simulink model "ds1_inter"  (R2019a)
settings: Solver=ode14x  StartTime=beginTime  StopTime=0.166  FixedStep=1e-4  RelTol=1e-3  EnableMultiTasking=on
model workspace (MAT data in the model file):
  Ankle_L_D = 0.125126243033
  Ankle_L_S = 0.0328154604487
  Ankle_R_D = 0.245807097642
  Ankle_R_S = 0.682954357178
  F_C = 0.06105
  F_H = 0.07
  F_I = 0.00125071180063
  F_L = 0.185
  F_M = 1.13129
  F_W = 0.1
  GRF_HD = 941.037069119
  GRF_HS = 1691.11560066
  GRF_VD = 12300.8672242
  GRF_VS = 71710.3574634
  HAT_I = 3.41998320224
  HAT_L = 0.51264
  HAT_M = 52.89756
  HAT_a = 0.2
  HAT_b = 0.11
  Hip_L_D = 0.0332143791481
  Hip_L_S = 0.0516603438036
  Hip_R_D = 0.145088103411
  Hip_R_S = 0.15911410017
  Knee_L_D = 0.0558982452805
  Knee_L_S = 0.00250387295429
  Knee_R_D = 0.0619293882143
  Knee_R_S = 0.0623339259595
  M : struct (value not decoded)
  Planar_joint_x_p_i = 0
  Planar_joint_x_v_i = 0.571578955042
  Planar_joint_y_p_i = 0
  Planar_joint_y_v_i = 0
  Planar_joint_z_p_i = 0
  Planar_joint_z_w_i = -47.4942945829
  S_I = 0.0556212184297
  S_L = 0.41
  S_M = 3.62793
  S_R1 = 0.035
  S_R2 = 0.0716197243914
  T_I = 0.63371745
  T_L = 0.6
  T_M = 7.802
  T_R1 = 0.0716197243914
  T_R2 = 0.105042262441
  beginTime = 0
  bodymass = 78.02
  lagStanceAnkle = [0 0 0 0 0 0]
  lagStanceKnee = [0 0 0 0 0 0]
  lagSwingAnkle = [0 0 0 0 0 0]
  lagSwingKnee = [0 0 0 0 0 0]
  p_stance_ankle_i = 12.5
  p_stance_hip_i = -24.9413676415
  p_stance_knee_i = -2.50807459996
  p_swing_ankle_i = 4.11757124464
  p_swing_hip_i = 18.3000604838
  p_swing_knee_i = -3.41741510381
  polyfit_stance_ankle = [-863347.977095 222377.922877 -7468.35453889 -9.40558010807 -153.06789694]
  polyfit_stance_hip = [-279786636.688 114363391.625 -15725654.0525 856134.662579 -22930.0516399 481.110496147 63.2694363354]
  polyfit_stance_knee = [-122862314.114 52903969.6705 -7988612.27678 487806.049871 -8969.32141641 330.337585729 -54.0526736443]
  polyfit_swing_ankle = [49510154320.8 -30205907167.6 7312588550.85 -888915044.437 56385922.5861 -1769074.37171 25613.4020917 -113.306543933 -1.03720591697]
  polyfit_swing_hip = [538683495113 -366532634246 101719653645 -14750073882.9 1184454520.37 -50949861.1242 1019832.60417 -6310.84925925 -38.0907282261]
  polyfit_swing_knee = [352478408737 -233011269241 62650744932.5 -8775138187.04 678489689.503 -28060179.8998 545151.783137 -3282.03325692 -26.455631467]
  time = [0 0.00833333333333 0.0166666666667 0.025 0.0333333333333 0.0416666666667 0.05 0.0583333333333 0.0666666666667 0.075 0.0833333333333 0.0916666666667 ... (21 elements, 21x1)]
  w_stance_ankle_i = 4.94863039576
  w_stance_hip_i = 2.61291825988
  w_stance_knee_i = 13.980565237
  w_swing_ankle_i = -56.5478745686
  w_swing_hip_i = 74.5733616561
  w_swing_knee_i = 18.8942606538
symbols that are objects in the model workspace (value not decoded): M
undefined symbols (not defined in the file): X, Y, Z
libraries: nesl_utility x101, sm_lib x68, fl_lib x24, fl_ps_legacy_lib x14, simulink x4
(part 4 of 8)

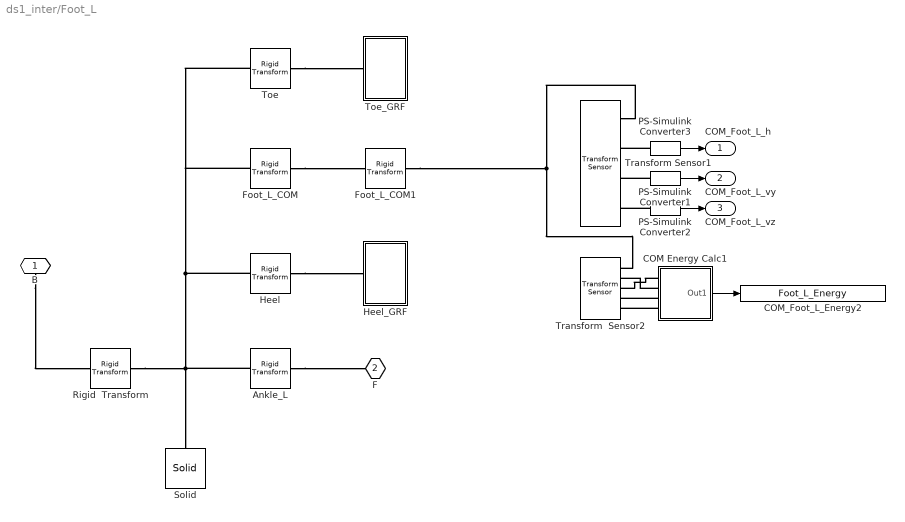
== system ds1_inter/Foot_L ==
  Ankle_L : sm_lib/Frames and Transforms/Rigid Transform  TranslationMethod=StandardAxis  TranslationStandardOffset=F_H  TranslationLengthUnit=m  TranslationStandardAxis=+Y  TranslationCartesianOffset=[0 0 0]  TranslationROffset=0  TranslationROffsetUnits=m  TranslationZOffset=0  TranslationZOffsetUnits=m  TranslationThetaOffset=0  TranslationThetaOffsetUnits=deg  RotationMethod=StandardAxis  RotationAngleUnits=deg  RotationStandardAxis=+Z  RotationAngle=-90  RotationArbitraryAxis=[0 0 1]  FollAlignAxisA=+Z  BaseAlignAxisA=+Z  FollAlignAxisB=+X  BaseAlignAxisB=+Y  RotationSequenceAxes=FollowerAxes  RotationSequence=XYX  RotationSequenceAngles=[0 0 0]  RotationSequenceAnglesUnits=deg  RotationMatrix=[1 0 0; 0 1 0; 0 0 1]
  COM Energy Calc1 : Subsystem
  COM_Foot_L_Energy2 : ToWorkspace  VariableName=Foot_L_Energy  SampleTime=-1
  Foot_L_COM : sm_lib/Frames and Transforms/Rigid Transform  TranslationMethod=StandardAxis  TranslationStandardOffset=(1/3)*F_H  TranslationLengthUnit=m  TranslationStandardAxis=+X  TranslationCartesianOffset=[0 0 0]  TranslationROffset=0  TranslationROffsetUnits=m  TranslationZOffset=0  TranslationZOffsetUnits=m  TranslationThetaOffset=0  TranslationThetaOffsetUnits=deg  RotationMethod=None  RotationAngleUnits=deg  RotationStandardAxis=+X  RotationAngle=0  RotationArbitraryAxis=[0 0 1]  FollAlignAxisA=+X  BaseAlignAxisA=+Z  FollAlignAxisB=+Y  BaseAlignAxisB=+X  RotationSequenceAxes=FollowerAxes  RotationSequence=XYX  RotationSequenceAngles=[0 0 0]  RotationSequenceAnglesUnits=deg  RotationMatrix=[1 0 0; 0 1 0; 0 0 1]
      settings: AttributesFormatString=|
      | {%<RotationStandardAxis>} %<RotationAngle> [%<RotationAngleUnits>]
      | {%<TranslationStandardAxis>} %<TranslationStandardOffset> [%<TranslationLengthUnit>]
  Foot_L_COM1 : sm_lib/Frames and Transforms/Rigid Transform  TranslationMethod=StandardAxis  TranslationStandardOffset=F_H/2  TranslationLengthUnit=m  TranslationStandardAxis=+Y  TranslationCartesianOffset=[0 0 0]  TranslationROffset=0  TranslationROffsetUnits=m  TranslationZOffset=0  TranslationZOffsetUnits=m  TranslationThetaOffset=0  TranslationThetaOffsetUnits=deg  RotationMethod=None  RotationAngleUnits=deg  RotationStandardAxis=+X  RotationAngle=(F_L-F_C)/2  RotationArbitraryAxis=[0 0 1]  FollAlignAxisA=+X  BaseAlignAxisA=+Z  FollAlignAxisB=+Y  BaseAlignAxisB=+X  RotationSequenceAxes=FollowerAxes  RotationSequence=XYX  RotationSequenceAngles=[0 0 0]  RotationSequenceAnglesUnits=deg  RotationMatrix=[1 0 0; 0 1 0; 0 0 1]
      settings: AttributesFormatString=|
      | {%<RotationStandardAxis>} %<RotationAngle> [%<RotationAngleUnits>]
      | {%<TranslationStandardAxis>} %<TranslationStandardOffset> [%<TranslationLengthUnit>]
  Heel : sm_lib/Frames and Transforms/Rigid Transform  TranslationMethod=StandardAxis  TranslationStandardOffset=F_C  TranslationLengthUnit=m  TranslationStandardAxis=-X  TranslationCartesianOffset=[0 0 0]  TranslationROffset=0  TranslationROffsetUnits=m  TranslationZOffset=0  TranslationZOffsetUnits=m  TranslationThetaOffset=0  TranslationThetaOffsetUnits=deg  RotationMethod=AlignedAxes  RotationAngleUnits=deg  RotationStandardAxis=+Z  RotationAngle=0  RotationArbitraryAxis=[0 0 1]  FollAlignAxisA=+X  BaseAlignAxisA=+Z  FollAlignAxisB=+Y  BaseAlignAxisB=+X  RotationSequenceAxes=FollowerAxes  RotationSequence=XYX  RotationSequenceAngles=[0 0 0]  RotationSequenceAnglesUnits=deg  RotationMatrix=[1 0 0; 0 1 0; 0 0 1]
  Heel_GRF : Subsystem
  PS-Simulink Converter1 : nesl_utility/PS-Simulink Converter  PhysicalDomain=network_engine_domain  SubClassName=ps_output  LeftPortType=input  RightPortType=output  PseudoPeriodic=off  Frequencies=[]  Unit=1  AffineConversion=off
  PS-Simulink Converter2 : nesl_utility/PS-Simulink Converter  PhysicalDomain=network_engine_domain  SubClassName=ps_output  LeftPortType=input  RightPortType=output  PseudoPeriodic=off  Frequencies=[]  Unit=1  AffineConversion=off
  PS-Simulink Converter3 : nesl_utility/PS-Simulink Converter  PhysicalDomain=network_engine_domain  SubClassName=ps_output  LeftPortType=input  RightPortType=output  PseudoPeriodic=off  Frequencies=[]  Unit=1  AffineConversion=off
  Rigid  Transform : sm_lib/Frames and Transforms/Rigid Transform  TranslationMethod=None  TranslationStandardOffset=T_R2  TranslationLengthUnit=m  TranslationStandardAxis=+Z  TranslationCartesianOffset=[0 0 0]  TranslationROffset=0  TranslationROffsetUnits=m  TranslationZOffset=0  TranslationZOffsetUnits=m  TranslationThetaOffset=0  TranslationThetaOffsetUnits=deg  RotationMethod=AlignedAxes  RotationAngleUnits=deg  RotationStandardAxis=+Z  RotationAngle=0  RotationArbitraryAxis=[0 0 1]  FollAlignAxisA=+X  BaseAlignAxisA=+Z  FollAlignAxisB=+Z  BaseAlignAxisB=+Y  RotationSequenceAxes=FollowerAxes  RotationSequence=XYX  RotationSequenceAngles=[0 0 0]  RotationSequenceAnglesUnits=deg  RotationMatrix=[1 0 0; 0 1 0; 0 0 1]
  Solid : sm_lib/Body Elements/Solid  InertiaType=Custom  Mass=F_M  MassUnits=kg  CenterOfMass=[(F_L-F_C)/2, F_H/2, 0]  CenterOfMassUnits=m  MomentsOfInertia=[0.001 0.001 F_I]  MomentsOfInertiaUnits=kg*m^2  ProductsOfInertia=[0 0 0]  ProductsOfInertiaUnits=kg*m^2  BasedOnType=Density  Density=0  DensityUnits=kg/(m^3)  DoExposeReferenceFrame=on  SerializedFrames=<Frames/>  GraphicType=FromGeometry  MarkerShape=Sphere  MarkerSize=10  MarkerSizeUnits=m  GraphicVisPropType=SimpleVisualProperties  GraphicDiffuseColor=[0.0 0.4 1.0]  GraphicSpecularColor=[0.5 0.5 0.5 1.0]  GraphicAmbientColor=[0.15 0.15 0.15 1.0]  GraphicEmissiveColor=[0.0 0.0 0.0 1.0]  GraphicShininess=75  GraphicOpacity=1.0  GeometryShape=GeneralExtrusion  RectangleSize=[1 1]  RectangleSizeUnits=m  BrickDimensions=[1 1 1]  BrickDimensionUnits=m  CylinderRadius=1  CylinderRadiusUnits=m  CylinderLength=1  CylinderLengthUnits=m  SphereRadius=1  SphereRadiusUnits=m  EllipsoidRadii=[1 1 1]  EllipsoidRadiiUnits=m  ExtrusionCrossSection=F_cross_section  ExtrusionCrossSectionUnits=m  ExtrusionLength=F_W  ExtrusionLengthUnits=m  PolygonNumSides=3  PolygonOuterRadius=1  PolygonOuterRadiusUnits=m  ExtGeomFileType=STEP  ExtGeomFileUnits=m  RevolutionCrossSection=[1 1; 1 -1; 2 -1; 2 1]  RevolutionCrossSectionUnits=m  RevolutionExtent=Full  RevolutionAngle=180  RevolutionAngleUnits=deg
  Toe : sm_lib/Frames and Transforms/Rigid Transform  TranslationMethod=StandardAxis  TranslationStandardOffset=F_L-F_C  TranslationLengthUnit=m  TranslationStandardAxis=+X  TranslationCartesianOffset=[0 0 0]  TranslationROffset=0  TranslationROffsetUnits=m  TranslationZOffset=0  TranslationZOffsetUnits=m  TranslationThetaOffset=0  TranslationThetaOffsetUnits=deg  RotationMethod=AlignedAxes  RotationAngleUnits=deg  RotationStandardAxis=+Z  RotationAngle=0  RotationArbitraryAxis=[0 0 1]  FollAlignAxisA=+X  BaseAlignAxisA=+Z  FollAlignAxisB=+Y  BaseAlignAxisB=+X  RotationSequenceAxes=FollowerAxes  RotationSequence=XYX  RotationSequenceAngles=[0 0 0]  RotationSequenceAnglesUnits=deg  RotationMatrix=[1 0 0; 0 1 0; 0 0 1]
  Toe_GRF : Subsystem
  Transform Sensor1 : sm_lib/Frames and Transforms/Transform Sensor  MeasurementFrame=World  SenseAngle=off  SenseAxis=off  SenseAngle1=off  SenseAngle2=off  SenseAngle3=off  SenseQ=off  SenseR=off  SenseOmegaX=off  SenseOmegaY=off  SenseOmegaZ=off  SenseOmega1=off  SenseOmega2=off  SenseOmega3=off  SenseQDot=off  SenseRDot=off  SenseAlphaX=off  SenseAlphaY=off  SenseAlphaZ=off  SenseAlpha1=off  SenseAlpha2=off  SenseAlpha3=off  SenseQDDot=off  SenseRDDot=off  SenseX=off  SenseY=off  SenseZ=on  SenseRad=off  SenseAzim=off  SenseDist=off  SenseInc=off  SenseXDot=off  SenseYDot=on  SenseZDot=on  SenseRadDot=off  SenseAzimDot=off  SenseDistDot=off  SenseIncDot=off  SenseXDDot=off  SenseYDDot=off  SenseZDDot=off  SenseRadDDot=off  SenseAzimDDot=off  SenseDistDDot=off  SenseIncDDot=off
  Transform  Sensor2 : sm_lib/Frames and Transforms/Transform Sensor  MeasurementFrame=World  SenseAngle=off  SenseAxis=off  SenseAngle1=off  SenseAngle2=off  SenseAngle3=off  SenseQ=off  SenseR=off  SenseOmegaX=on  SenseOmegaY=off  SenseOmegaZ=off  SenseOmega1=off  SenseOmega2=off  SenseOmega3=off  SenseQDot=off  SenseRDot=off  SenseAlphaX=off  SenseAlphaY=off  SenseAlphaZ=off  SenseAlpha1=off  SenseAlpha2=off  SenseAlpha3=off  SenseQDDot=off  SenseRDDot=off  SenseX=off  SenseY=off  SenseZ=on  SenseRad=off  SenseAzim=off  SenseDist=off  SenseInc=off  SenseXDot=off  SenseYDot=on  SenseZDot=on  SenseRadDot=off  SenseAzimDot=off  SenseDistDot=off  SenseIncDot=off  SenseXDDot=off  SenseYDDot=off  SenseZDDot=off  SenseRadDDot=off  SenseAzimDDot=off  SenseDistDDot=off  SenseIncDDot=off
  B : PMIOPort  Side=Right
  F : PMIOPort  Port=2  Side=Left
  " COM_Foot_L_h" : Outport
  " COM_Foot_L_vy" : Outport  Port=2
  " COM_Foot_L_vz" : Outport  Port=3
  wires:
  COM Energy Calc1/1(Out1) -> COM_Foot_L_Energy2/1
  PS-Simulink Converter1/1 -> " COM_Foot_L_vy"/1
  PS-Simulink Converter3/1 -> " COM_Foot_L_h"/1
  PS-Simulink Converter2/1 -> " COM_Foot_L_vz"/1
  connections:
  B/RConn1 -- Rigid  Transform/RConn1
  Rigid  Transform/LConn1 -- Ankle_L/LConn1 -- Foot_L_COM/LConn1 -- Toe/LConn1 -- Heel/LConn1 -- Solid/RConn1
  Ankle_L/RConn1 -- F/RConn1
  Toe/RConn1 -- Toe_GRF/LConn1
  Heel/RConn1 -- Heel_GRF/LConn1
  Transform Sensor1/RConn1 -- Transform  Sensor2/RConn1 -- Foot_L_COM1/RConn1
  COM Energy Calc1/LConn2 -- Transform  Sensor2/RConn2
  COM Energy Calc1/LConn4 -- Transform  Sensor2/RConn5
  PS-Simulink Converter1/LConn1 -- Transform Sensor1/RConn3
  COM Energy Calc1/LConn1 -- Transform  Sensor2/RConn3
  PS-Simulink Converter2/LConn1 -- Transform Sensor1/RConn4
  COM Energy Calc1/LConn3 -- Transform  Sensor2/RConn4
  PS-Simulink Converter3/LConn1 -- Transform Sensor1/RConn2
  Foot_L_COM/RConn1 -- Foot_L_COM1/LConn1

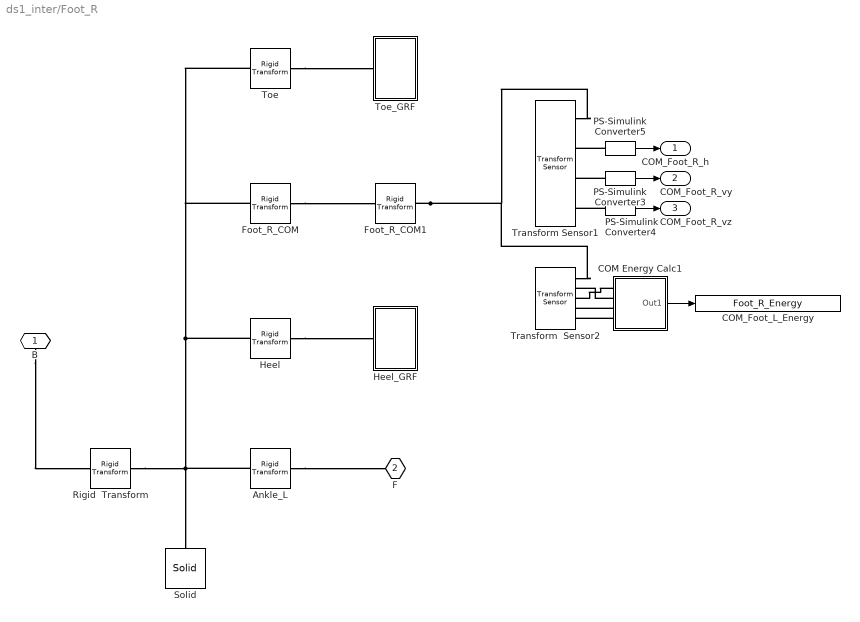
== system ds1_inter/Foot_R ==
  Ankle_L : sm_lib/Frames and Transforms/Rigid Transform  TranslationMethod=StandardAxis  TranslationStandardOffset=F_H  TranslationLengthUnit=m  TranslationStandardAxis=+Y  TranslationCartesianOffset=[0 0 0]  TranslationROffset=0  TranslationROffsetUnits=m  TranslationZOffset=0  TranslationZOffsetUnits=m  TranslationThetaOffset=0  TranslationThetaOffsetUnits=deg  RotationMethod=StandardAxis  RotationAngleUnits=deg  RotationStandardAxis=+Z  RotationAngle=-90  RotationArbitraryAxis=[0 0 1]  FollAlignAxisA=+Z  BaseAlignAxisA=+Z  FollAlignAxisB=+X  BaseAlignAxisB=+Y  RotationSequenceAxes=FollowerAxes  RotationSequence=XYX  RotationSequenceAngles=[0 0 0]  RotationSequenceAnglesUnits=deg  RotationMatrix=[1 0 0; 0 1 0; 0 0 1]
      settings: AttributesFormatString=|
      | {%<RotationStandardAxis>} %<RotationAngle> [%<RotationAngleUnits>]
      | {%<TranslationStandardAxis>} %<TranslationStandardOffset> [%<TranslationLengthUnit>]
  COM Energy Calc1 : Subsystem
  COM_Foot_L_Energy : ToWorkspace  VariableName=Foot_R_Energy  SampleTime=-1
  Foot_R_COM : sm_lib/Frames and Transforms/Rigid Transform  TranslationMethod=StandardAxis  TranslationStandardOffset=(1/3)*F_H  TranslationLengthUnit=m  TranslationStandardAxis=+X  TranslationCartesianOffset=[0 0 0]  TranslationROffset=0  TranslationROffsetUnits=m  TranslationZOffset=0  TranslationZOffsetUnits=m  TranslationThetaOffset=0  TranslationThetaOffsetUnits=deg  RotationMethod=None  RotationAngleUnits=deg  RotationStandardAxis=+X  RotationAngle=0  RotationArbitraryAxis=[0 0 1]  FollAlignAxisA=+X  BaseAlignAxisA=+Z  FollAlignAxisB=+Y  BaseAlignAxisB=+X  RotationSequenceAxes=FollowerAxes  RotationSequence=XYX  RotationSequenceAngles=[0 0 0]  RotationSequenceAnglesUnits=deg  RotationMatrix=[1 0 0; 0 1 0; 0 0 1]
      settings: AttributesFormatString=|
      | {%<RotationStandardAxis>} %<RotationAngle> [%<RotationAngleUnits>]
      | {%<TranslationStandardAxis>} %<TranslationStandardOffset> [%<TranslationLengthUnit>]
  Foot_R_COM1 : sm_lib/Frames and Transforms/Rigid Transform  TranslationMethod=StandardAxis  TranslationStandardOffset=F_H/2  TranslationLengthUnit=m  TranslationStandardAxis=+Y  TranslationCartesianOffset=[0 0 0]  TranslationROffset=0  TranslationROffsetUnits=m  TranslationZOffset=0  TranslationZOffsetUnits=m  TranslationThetaOffset=0  TranslationThetaOffsetUnits=deg  RotationMethod=None  RotationAngleUnits=deg  RotationStandardAxis=+X  RotationAngle=(F_L-F_C)/2  RotationArbitraryAxis=[0 0 1]  FollAlignAxisA=+X  BaseAlignAxisA=+Z  FollAlignAxisB=+Y  BaseAlignAxisB=+X  RotationSequenceAxes=FollowerAxes  RotationSequence=XYX  RotationSequenceAngles=[0 0 0]  RotationSequenceAnglesUnits=deg  RotationMatrix=[1 0 0; 0 1 0; 0 0 1]
      settings: AttributesFormatString=|
      | {%<RotationStandardAxis>} %<RotationAngle> [%<RotationAngleUnits>]
      | {%<TranslationStandardAxis>} %<TranslationStandardOffset> [%<TranslationLengthUnit>]
  Heel : sm_lib/Frames and Transforms/Rigid Transform  TranslationMethod=StandardAxis  TranslationStandardOffset=F_C  TranslationLengthUnit=m  TranslationStandardAxis=-X  TranslationCartesianOffset=[0 0 0]  TranslationROffset=0  TranslationROffsetUnits=m  TranslationZOffset=0  TranslationZOffsetUnits=m  TranslationThetaOffset=0  TranslationThetaOffsetUnits=deg  RotationMethod=AlignedAxes  RotationAngleUnits=deg  RotationStandardAxis=+Z  RotationAngle=0  RotationArbitraryAxis=[0 0 1]  FollAlignAxisA=+X  BaseAlignAxisA=+Z  FollAlignAxisB=+Y  BaseAlignAxisB=+X  RotationSequenceAxes=FollowerAxes  RotationSequence=XYX  RotationSequenceAngles=[0 0 0]  RotationSequenceAnglesUnits=deg  RotationMatrix=[1 0 0; 0 1 0; 0 0 1]
      settings: AttributesFormatString=|
      | {%<RotationStandardAxis>} %<RotationAngle> [%<RotationAngleUnits>]
      | {%<TranslationStandardAxis>} %<TranslationStandardOffset> [%<TranslationLengthUnit>]
  Heel_GRF : Subsystem
  PS-Simulink Converter3 : nesl_utility/PS-Simulink Converter  PhysicalDomain=network_engine_domain  SubClassName=ps_output  LeftPortType=input  RightPortType=output  PseudoPeriodic=off  Frequencies=[]  Unit=1  AffineConversion=off
  PS-Simulink Converter4 : nesl_utility/PS-Simulink Converter  PhysicalDomain=network_engine_domain  SubClassName=ps_output  LeftPortType=input  RightPortType=output  PseudoPeriodic=off  Frequencies=[]  Unit=1  AffineConversion=off
  PS-Simulink Converter5 : nesl_utility/PS-Simulink Converter  PhysicalDomain=network_engine_domain  SubClassName=ps_output  LeftPortType=input  RightPortType=output  PseudoPeriodic=off  Frequencies=[]  Unit=1  AffineConversion=off
  Rigid  Transform : sm_lib/Frames and Transforms/Rigid Transform  TranslationMethod=StandardAxis  TranslationStandardOffset=T_R2  TranslationLengthUnit=m  TranslationStandardAxis=+Z  TranslationCartesianOffset=[0 0 0]  TranslationROffset=0  TranslationROffsetUnits=m  TranslationZOffset=0  TranslationZOffsetUnits=m  TranslationThetaOffset=0  TranslationThetaOffsetUnits=deg  RotationMethod=AlignedAxes  RotationAngleUnits=deg  RotationStandardAxis=+Z  RotationAngle=0  RotationArbitraryAxis=[0 0 1]  FollAlignAxisA=+X  BaseAlignAxisA=+Z  FollAlignAxisB=+Z  BaseAlignAxisB=+Y  RotationSequenceAxes=FollowerAxes  RotationSequence=XYX  RotationSequenceAngles=[0 0 0]  RotationSequenceAnglesUnits=deg  RotationMatrix=[1 0 0; 0 1 0; 0 0 1]
      settings: AttributesFormatString=|
      | {%<RotationStandardAxis>} %<RotationAngle> [%<RotationAngleUnits>]
      | {%<TranslationStandardAxis>} %<TranslationStandardOffset> [%<TranslationLengthUnit>]
  Solid : sm_lib/Body Elements/Solid  InertiaType=Custom  Mass=F_M  MassUnits=kg  CenterOfMass=[(F_L-F_C)/2, F_H/2, 0]  CenterOfMassUnits=m  MomentsOfInertia=[0.001 0.001 F_I]  MomentsOfInertiaUnits=kg*m^2  ProductsOfInertia=[0 0 0]  ProductsOfInertiaUnits=kg*m^2  BasedOnType=Density  Density=0  DensityUnits=kg/(m^3)  DoExposeReferenceFrame=on  SerializedFrames=<Frames/>  GraphicType=FromGeometry  MarkerShape=Sphere  MarkerSize=10  MarkerSizeUnits=m  GraphicVisPropType=SimpleVisualProperties  GraphicDiffuseColor=[0.0 0.4 1.0]  GraphicSpecularColor=[0.5 0.5 0.5 1.0]  GraphicAmbientColor=[0.15 0.15 0.15 1.0]  GraphicEmissiveColor=[0.0 0.0 0.0 1.0]  GraphicShininess=75  GraphicOpacity=1.0  GeometryShape=GeneralExtrusion  RectangleSize=[1 1]  RectangleSizeUnits=m  BrickDimensions=[1 1 1]  BrickDimensionUnits=m  CylinderRadius=1  CylinderRadiusUnits=m  CylinderLength=1  CylinderLengthUnits=m  SphereRadius=1  SphereRadiusUnits=m  EllipsoidRadii=[1 1 1]  EllipsoidRadiiUnits=m  ExtrusionCrossSection=F_cross_section  ExtrusionCrossSectionUnits=m  ExtrusionLength=F_W  ExtrusionLengthUnits=m  PolygonNumSides=3  PolygonOuterRadius=1  PolygonOuterRadiusUnits=m  ExtGeomFileType=STEP  ExtGeomFileUnits=m  RevolutionCrossSection=[1 1; 1 -1; 2 -1; 2 1]  RevolutionCrossSectionUnits=m  RevolutionExtent=Full  RevolutionAngle=180  RevolutionAngleUnits=deg
  Toe : sm_lib/Frames and Transforms/Rigid Transform  TranslationMethod=StandardAxis  TranslationStandardOffset=F_L-F_C  TranslationLengthUnit=m  TranslationStandardAxis=+X  TranslationCartesianOffset=[0 0 0]  TranslationROffset=0  TranslationROffsetUnits=m  TranslationZOffset=0  TranslationZOffsetUnits=m  TranslationThetaOffset=0  TranslationThetaOffsetUnits=deg  RotationMethod=AlignedAxes  RotationAngleUnits=deg  RotationStandardAxis=+Z  RotationAngle=0  RotationArbitraryAxis=[0 0 1]  FollAlignAxisA=+X  BaseAlignAxisA=+Z  FollAlignAxisB=+Y  BaseAlignAxisB=+X  RotationSequenceAxes=FollowerAxes  RotationSequence=XYX  RotationSequenceAngles=[0 0 0]  RotationSequenceAnglesUnits=deg  RotationMatrix=[1 0 0; 0 1 0; 0 0 1]
      settings: AttributesFormatString=|
      | {%<RotationStandardAxis>} %<RotationAngle> [%<RotationAngleUnits>]
      | {%<TranslationStandardAxis>} %<TranslationStandardOffset> [%<TranslationLengthUnit>]
  "Toe_GRF " : Subsystem
  Transform Sensor1 : sm_lib/Frames and Transforms/Transform Sensor  MeasurementFrame=World  SenseAngle=off  SenseAxis=off  SenseAngle1=off  SenseAngle2=off  SenseAngle3=off  SenseQ=off  SenseR=off  SenseOmegaX=off  SenseOmegaY=off  SenseOmegaZ=off  SenseOmega1=off  SenseOmega2=off  SenseOmega3=off  SenseQDot=off  SenseRDot=off  SenseAlphaX=off  SenseAlphaY=off  SenseAlphaZ=off  SenseAlpha1=off  SenseAlpha2=off  SenseAlpha3=off  SenseQDDot=off  SenseRDDot=off  SenseX=off  SenseY=off  SenseZ=on  SenseRad=off  SenseAzim=off  SenseDist=off  SenseInc=off  SenseXDot=off  SenseYDot=on  SenseZDot=on  SenseRadDot=off  SenseAzimDot=off  SenseDistDot=off  SenseIncDot=off  SenseXDDot=off  SenseYDDot=off  SenseZDDot=off  SenseRadDDot=off  SenseAzimDDot=off  SenseDistDDot=off  SenseIncDDot=off
  Transform  Sensor2 : sm_lib/Frames and Transforms/Transform Sensor  MeasurementFrame=World  SenseAngle=off  SenseAxis=off  SenseAngle1=off  SenseAngle2=off  SenseAngle3=off  SenseQ=off  SenseR=off  SenseOmegaX=on  SenseOmegaY=off  SenseOmegaZ=off  SenseOmega1=off  SenseOmega2=off  SenseOmega3=off  SenseQDot=off  SenseRDot=off  SenseAlphaX=off  SenseAlphaY=off  SenseAlphaZ=off  SenseAlpha1=off  SenseAlpha2=off  SenseAlpha3=off  SenseQDDot=off  SenseRDDot=off  SenseX=off  SenseY=off  SenseZ=on  SenseRad=off  SenseAzim=off  SenseDist=off  SenseInc=off  SenseXDot=off  SenseYDot=on  SenseZDot=on  SenseRadDot=off  SenseAzimDot=off  SenseDistDot=off  SenseIncDot=off  SenseXDDot=off  SenseYDDot=off  SenseZDDot=off  SenseRadDDot=off  SenseAzimDDot=off  SenseDistDDot=off  SenseIncDDot=off
  B : PMIOPort  Side=Right
  F : PMIOPort  Port=2  Side=Left
  COM_Foot_R_h : Outport
  COM_Foot_R_vy : Outport  Port=2
  COM_Foot_R_vz : Outport  Port=3
  wires:
  PS-Simulink Converter5/1 -> COM_Foot_R_h/1
  PS-Simulink Converter4/1 -> COM_Foot_R_vz/1
  COM Energy Calc1/1(Out1) -> COM_Foot_L_Energy/1
  PS-Simulink Converter3/1 -> COM_Foot_R_vy/1
  connections:
  B/RConn1 -- Rigid  Transform/RConn1
  Rigid  Transform/LConn1 -- Ankle_L/LConn1 -- Foot_R_COM/LConn1 -- Toe/LConn1 -- Heel/LConn1 -- Solid/RConn1
  Ankle_L/RConn1 -- F/RConn1
  Heel/RConn1 -- Heel_GRF/LConn1
  Toe/RConn1 -- "Toe_GRF "/LConn1
  Foot_R_COM1/RConn1 -- Transform  Sensor2/RConn1 -- Transform Sensor1/RConn1
  PS-Simulink Converter5/LConn1 -- Transform Sensor1/RConn2
  COM Energy Calc1/LConn1 -- Transform  Sensor2/RConn3
  COM Energy Calc1/LConn2 -- Transform  Sensor2/RConn2
  COM Energy Calc1/LConn4 -- Transform  Sensor2/RConn5
  COM Energy Calc1/LConn3 -- Transform  Sensor2/RConn4
  PS-Simulink Converter4/LConn1 -- Transform Sensor1/RConn4
  PS-Simulink Converter3/LConn1 -- Transform Sensor1/RConn3
  Foot_R_COM/RConn1 -- Foot_R_COM1/LConn1

== system ds1_inter/HAT ==
  note: %vCOMCal  uses transform sensor to read velocity of COM in y(forward)
      | and z(up) wrt world frame
  Gain : Gain  Gain=180/pi
  PS-Simulink Converter{,1..3} (4 alike) : nesl_utility/PS-Simulink Converter  PhysicalDomain=network_engine_domain  SubClassName=ps_output  LeftPortType=input  RightPortType=output  PseudoPeriodic=off  Frequencies=[]  Unit=1  AffineConversion=off
  PredictedCOMVelocity_y : ToWorkspace  VariableName=PredictedCOMVelocity_y  SampleTime=-1
      settings: MaxDataPoints=1  Decimation=3
  PredictedCOMVelocity_y1 : ToWorkspace  VariableName=PredictedCOMVelocity_z  SampleTime=-1
      settings: MaxDataPoints=1  Decimation=3
  Rigid  Transform : sm_lib/Frames and Transforms/Rigid Transform  TranslationMethod=Cartesian  TranslationStandardOffset=0  TranslationLengthUnit=m  TranslationStandardAxis=+Z  TranslationCartesianOffset=[-T_R2, 0, -HAT_L/2]  TranslationROffset=0  TranslationROffsetUnits=m  TranslationZOffset=0  TranslationZOffsetUnits=m  TranslationThetaOffset=0  TranslationThetaOffsetUnits=deg  RotationMethod=StandardAxis  RotationAngleUnits=deg  RotationStandardAxis=+Y  RotationAngle=90  RotationArbitraryAxis=[0 0 1]  FollAlignAxisA=+X  BaseAlignAxisA=+Y  FollAlignAxisB=+Y  BaseAlignAxisB=+Z  RotationSequenceAxes=FollowerAxes  RotationSequence=XYX  RotationSequenceAngles=[0 0 0]  RotationSequenceAnglesUnits=deg  RotationMatrix=[1 0 0; 0 1 0; 0 0 1]
  Rigid  Transform1 : sm_lib/Frames and Transforms/Rigid Transform  TranslationMethod=Cartesian  TranslationStandardOffset=0  TranslationLengthUnit=m  TranslationStandardAxis=+Z  TranslationCartesianOffset=[T_R2, 0, -HAT_L/2]  TranslationROffset=0  TranslationROffsetUnits=m  TranslationZOffset=0  TranslationZOffsetUnits=m  TranslationThetaOffset=0  TranslationThetaOffsetUnits=deg  RotationMethod=StandardAxis  RotationAngleUnits=deg  RotationStandardAxis=+Y  RotationAngle=90  RotationArbitraryAxis=[0 0 1]  FollAlignAxisA=+X  BaseAlignAxisA=+Y  FollAlignAxisB=+Y  BaseAlignAxisB=+Z  RotationSequenceAxes=FollowerAxes  RotationSequence=XYX  RotationSequenceAngles=[0 0 0]  RotationSequenceAnglesUnits=deg  RotationMatrix=[1 0 0; 0 1 0; 0 0 1]
  Scope : Scope
  Scope1 : Scope
  Scope2 : Scope
  Solid : sm_lib/Body Elements/Solid  InertiaType=Custom  Mass=HAT_M  MassUnits=kg  CenterOfMass=[0 0 .126*HAT_L]  CenterOfMassUnits=m  MomentsOfInertia=[HAT_I .001 .001]  MomentsOfInertiaUnits=kg*m^2  ProductsOfInertia=[0 0 0]  ProductsOfInertiaUnits=kg*m^2  BasedOnType=Density  Density=1000  DensityUnits=kg/(m^3)  DoExposeReferenceFrame=on  SerializedFrames=<Frames/>  GraphicType=FromGeometry  MarkerShape=Sphere  MarkerSize=10  MarkerSizeUnits=m  GraphicVisPropType=SimpleVisualProperties  GraphicDiffuseColor=[0.0 0.4 1.0]  GraphicSpecularColor=[0.5 0.5 0.5 1.0]  GraphicAmbientColor=[0.15 0.15 0.15 1.0]  GraphicEmissiveColor=[0.0 0.0 0.0 1.0]  GraphicShininess=75  GraphicOpacity=1.0  GeometryShape=GeneralExtrusion  RectangleSize=[1 1]  RectangleSizeUnits=m  BrickDimensions=[1 1 1]  BrickDimensionUnits=m  CylinderRadius=1  CylinderRadiusUnits=m  CylinderLength=1  CylinderLengthUnits=m  SphereRadius=1  SphereRadiusUnits=m  EllipsoidRadii=[1 1 1]  EllipsoidRadiiUnits=m  ExtrusionCrossSection=HAT_cross_section  ExtrusionCrossSectionUnits=m  ExtrusionLength=HAT_L  ExtrusionLengthUnits=m  PolygonNumSides=3  PolygonOuterRadius=1  PolygonOuterRadiusUnits=m  ExtGeomFileType=STEP  ExtGeomFileUnits=m  RevolutionCrossSection=[1 1; 1 -1; 2 -1; 2 1]  RevolutionCrossSectionUnits=m  RevolutionExtent=Full  RevolutionAngle=180  RevolutionAngleUnits=deg
  Transform  Sensor : sm_lib/Frames and Transforms/Transform Sensor  MeasurementFrame=World  SenseAngle=on  SenseAxis=off  SenseAngle1=off  SenseAngle2=off  SenseAngle3=off  SenseQ=off  SenseR=off  SenseOmegaX=off  SenseOmegaY=off  SenseOmegaZ=off  SenseOmega1=off  SenseOmega2=off  SenseOmega3=off  SenseQDot=off  SenseRDot=off  SenseAlphaX=off  SenseAlphaY=off  SenseAlphaZ=off  SenseAlpha1=off  SenseAlpha2=off  SenseAlpha3=off  SenseQDDot=off  SenseRDDot=off  SenseX=off  SenseY=off  SenseZ=off  SenseRad=off  SenseAzim=off  SenseDist=off  SenseInc=off  SenseXDot=on  SenseYDot=on  SenseZDot=on  SenseRadDot=off  SenseAzimDot=off  SenseDistDot=off  SenseIncDot=off  SenseXDDot=off  SenseYDDot=off  SenseZDDot=off  SenseRadDDot=off  SenseAzimDDot=off  SenseDistDDot=off  SenseIncDDot=off
  vCOMCal : Subsystem
  B : PMIOPort  Side=Right
  F1 : PMIOPort  Port=2  Side=Left
  F2 : PMIOPort  Port=3  Side=Left
  HAT_position : Outport
  wires:
  PS-Simulink Converter/1 -> Gain/1
  Gain/1 -> HAT_position/1
  PS-Simulink Converter1/1 -> Scope/1
  PS-Simulink Converter2/1 -> Scope1/1
  PS-Simulink Converter3/1 -> Scope2/1
  vCOMCal/2(vCOM_z) -> PredictedCOMVelocity_y1/1
  vCOMCal/1(vCOM_y) -> PredictedCOMVelocity_y/1
  connections:
  B/RConn1 -- Transform  Sensor/RConn1 -- Rigid  Transform1/LConn1 -- Solid/RConn1 -- Rigid  Transform/LConn1
  Rigid  Transform1/RConn1 -- F2/RConn1
  Rigid  Transform/RConn1 -- vCOMCal/LConn1 -- F1/RConn1
  Transform  Sensor/RConn2 -- PS-Simulink Converter/LConn1
  Transform  Sensor/RConn3 -- PS-Simulink Converter1/LConn1
  Transform  Sensor/RConn4 -- PS-Simulink Converter2/LConn1
  Transform  Sensor/RConn5 -- PS-Simulink Converter3/LConn1

== system ds1_inter/Hip_L_Actuation ==
  Clock : Clock
  Gain : Gain  Gain=-1
  Hard_Stop_Hip_L : Subsystem  mask{upper_bound=((125-p_stance_hip_i)*pi)/180, lower_bound=((-30-p_stance_hip_i)*pi)/180, contact_stiffness=1e8, contact_damping=5000, initial_angular_position=0}
      mask prompts: upper_bound "Upper Bound"; lower_bound "Lower Bound"; contact_stiffness "Contact Stiffness"; contact_damping "Contact Damping"; initial_angular_position "Initial Angular Position"
  Hip_D_lookup : Lookup_n-D  NumberOfTableDimensions=1  BreakpointsForDimension1=[-30:.01:125]  Table=[exp(linspace(log(1000),log(.01),1000)), zeros(1,13500),exp(linspace(log(.01),log(1000),1001))]  RndMeth=Simplest  InputSameDT=on
  Hip_S_lookup : Lookup_n-D  NumberOfTableDimensions=1  BreakpointsForDimension1=[-30:.01:125]  Table=[exp(linspace(log(10000),log(.01),1000)), zeros(1,13500),exp(linspace(log(.01),log(10000),1001))]  RndMeth=Simplest  InputSameDT=on
  PS Add : fl_ps_legacy_lib/Legacy Physical Signals/Functions/PS Add
      settings: SourceProductName=Simscape  SourceProductBaseCode=SS
  PS Add1 : fl_ps_legacy_lib/Legacy Physical Signals/Functions/PS Add
      settings: SourceProductName=Simscape  SourceProductBaseCode=SS
  PS Lookup Table (1D) : fl_ps_legacy_lib/Legacy Physical Signals/Lookup Tables/PS Lookup Table (1D)  x=linspace(0,.1667,21)'  f=(-M.stance_hip/1000)*bodymass  interp_method=2  extrap_method=1
      settings: SourceProductName=Simscape  SourceProductBaseCode=SS
  PS-Simulink Converter1 : nesl_utility/PS-Simulink Converter  PhysicalDomain=network_engine_domain  SubClassName=ps_output  LeftPortType=input  RightPortType=output  PseudoPeriodic=off  Frequencies=[]  Unit=1  AffineConversion=off
  PS-Simulink Converter2 : nesl_utility/PS-Simulink Converter  PhysicalDomain=network_engine_domain  SubClassName=ps_output  LeftPortType=input  RightPortType=output  PseudoPeriodic=off  Frequencies=[]  Unit=1  AffineConversion=off
  Product : Product  RndMeth=Zero
  Product1 : Product  RndMeth=Zero
  Simulink-PS Converter : nesl_utility/Simulink-PS Converter  PhysicalDomain=network_engine_domain  SubClassName=ps_input  LeftPortType=input  RightPortType=output  PseudoPeriodic=off  Frequencies=[]  NoiseDistribution=none  NoiseParameters=[]  Unit=1  AffineConversion=off  FilteringAndDerivatives=zero  SimscapeFilterOrder=1  InputFilterTimeConstant=.001  UdotUserProvided=[]
  Simulink-PS Converter1 : nesl_utility/Simulink-PS Converter  PhysicalDomain=network_engine_domain  SubClassName=ps_input  LeftPortType=input  RightPortType=output  PseudoPeriodic=off  Frequencies=[]  NoiseDistribution=none  NoiseParameters=[]  Unit=1  AffineConversion=off  FilteringAndDerivatives=zero  SimscapeFilterOrder=1  InputFilterTimeConstant=.001  UdotUserProvided=[]
  Sum : Sum  Inputs=|++
  rad2deg : Gain  Gain=180/pi
  "rad2deg1 " : Gain  Gain=180/pi
  w : PMIOPort  Side=Right
  t : PMIOPort  Port=2  Side=Left
  q : PMIOPort  Port=3  Side=Right
  wires:
  PS-Simulink Converter1/1 -> "rad2deg1 "/1
  PS-Simulink Converter2/1 -> rad2deg/1
  rad2deg/1 -> Hip_S_lookup/1, Hip_D_lookup/1, Product/2
  Hip_S_lookup/1 -> Product/1
  "rad2deg1 "/1 -> Product1/1
  Product1/1 -> Sum/1
  Product/1 -> Sum/2
  Sum/1 -> Gain/1
  Gain/1 -> Simulink-PS Converter1/1
  Hip_D_lookup/1 -> Product1/2
  Clock/1 -> Simulink-PS Converter/1
  connections:
  w/RConn1 -- PS-Simulink Converter1/LConn1 -- Hard_Stop_Hip_L/LConn1
  Hard_Stop_Hip_L/RConn1 -- PS Add/LConn2
  q/RConn1 -- PS-Simulink Converter2/LConn1
  PS Add1/RConn1 -- t/RConn1
  PS Add/RConn1 -- PS Add1/LConn1
  Simulink-PS Converter1/RConn1 -- PS Add1/LConn2
  PS Lookup Table (1D)/RConn1 -- PS Add/LConn1
  Simulink-PS Converter/RConn1 -- PS Lookup Table (1D)/LConn1

== system ds1_inter/Hip_R_Actuation ==
  Clock : Clock
  Gain : Gain  Gain=-1
  Hard_Stop_Hip_R : Subsystem  mask{upper_bound=((125-p_swing_hip_i)*pi)/180, lower_bound=((-30-p_swing_hip_i)*pi)/180, contact_stiffness=1e8, contact_damping=5000, initial_angular_position=0}
      mask prompts: upper_bound "Upper Bound"; lower_bound "Lower Bound"; contact_stiffness "Contact Stiffness"; contact_damping "Contact Damping"; initial_angular_position "Initial Angular Position"
  Hip_D_lookup : Lookup_n-D  NumberOfTableDimensions=1  BreakpointsForDimension1=[-30:.01:125]  Table=[exp(linspace(log(1000),log(.01),1000)), zeros(1,13500),exp(linspace(log(.01),log(1000),1001))]  RndMeth=Simplest  InputSameDT=on
  Hip_S_lookup : Lookup_n-D  NumberOfTableDimensions=1  BreakpointsForDimension1=[-30:.01:125]  Table=[exp(linspace(log(10000),log(.01),1000)), zeros(1,13500),exp(linspace(log(.01),log(10000),1001))]  RndMeth=Simplest  InputSameDT=on
  PS Add : fl_ps_legacy_lib/Legacy Physical Signals/Functions/PS Add
      settings: SourceProductName=Simscape  SourceProductBaseCode=SS
  PS Add1 : fl_ps_legacy_lib/Legacy Physical Signals/Functions/PS Add
      settings: SourceProductName=Simscape  SourceProductBaseCode=SS
  PS Lookup Table (1D) : fl_ps_legacy_lib/Legacy Physical Signals/Lookup Tables/PS Lookup Table (1D)  x=linspace(0,.1667,21)'  f=(-M.strike_hip/1000)*bodymass  interp_method=2  extrap_method=1
      settings: SourceProductName=Simscape  SourceProductBaseCode=SS
  PS-Simulink Converter1 : nesl_utility/PS-Simulink Converter  PhysicalDomain=network_engine_domain  SubClassName=ps_output  LeftPortType=input  RightPortType=output  PseudoPeriodic=off  Frequencies=[]  Unit=1  AffineConversion=off
  PS-Simulink Converter2 : nesl_utility/PS-Simulink Converter  PhysicalDomain=network_engine_domain  SubClassName=ps_output  LeftPortType=input  RightPortType=output  PseudoPeriodic=off  Frequencies=[]  Unit=1  AffineConversion=off
  Product : Product  RndMeth=Zero
  Product1 : Product  RndMeth=Zero
  Simulink-PS Converter : nesl_utility/Simulink-PS Converter  PhysicalDomain=network_engine_domain  SubClassName=ps_input  LeftPortType=input  RightPortType=output  PseudoPeriodic=off  Frequencies=[]  NoiseDistribution=none  NoiseParameters=[]  Unit=1  AffineConversion=off  FilteringAndDerivatives=zero  SimscapeFilterOrder=1  InputFilterTimeConstant=.001  UdotUserProvided=[]
  Simulink-PS Converter1 : nesl_utility/Simulink-PS Converter  PhysicalDomain=network_engine_domain  SubClassName=ps_input  LeftPortType=input  RightPortType=output  PseudoPeriodic=off  Frequencies=[]  NoiseDistribution=none  NoiseParameters=[]  Unit=1  AffineConversion=off  FilteringAndDerivatives=zero  SimscapeFilterOrder=1  InputFilterTimeConstant=.001  UdotUserProvided=[]
  Sum : Sum  Inputs=|++
  rad2deg : Gain  Gain=180/pi
  "rad2deg1 " : Gain  Gain=180/pi
  w : PMIOPort  Side=Right
  t : PMIOPort  Port=2  Side=Left
  q : PMIOPort  Port=3  Side=Right
  wires:
  Clock/1 -> Simulink-PS Converter/1
  PS-Simulink Converter1/1 -> "rad2deg1 "/1
  PS-Simulink Converter2/1 -> rad2deg/1
  rad2deg/1 -> Hip_S_lookup/1, Hip_D_lookup/1, Product/2
  Hip_S_lookup/1 -> Product/1
  "rad2deg1 "/1 -> Product1/1
  Product1/1 -> Sum/1
  Product/1 -> Sum/2
  Sum/1 -> Gain/1
  Gain/1 -> Simulink-PS Converter1/1
  Hip_D_lookup/1 -> Product1/2
  connections:
  Hard_Stop_Hip_R/RConn1 -- PS Add/LConn2
  Hard_Stop_Hip_R/LConn1 -- PS-Simulink Converter1/LConn1 -- w/RConn1
  Simulink-PS Converter/RConn1 -- PS Lookup Table (1D)/LConn1
  q/RConn1 -- PS-Simulink Converter2/LConn1
  PS Add/RConn1 -- PS Add1/LConn1
  PS Add1/RConn1 -- t/RConn1
  PS Lookup Table (1D)/RConn1 -- PS Add/LConn1
  Simulink-PS Converter1/RConn1 -- PS Add1/LConn2
